simulink model "ModelOfOven"  (R2015a)
settings: Solver=ode3  StartTime=0.0  StopTime=1450  RelTol=1e-3
undefined symbols (not defined in the file or in its folder): sigbuilder_block
libraries: simulink x2, fuzblock x1, sldrtlib x1
settings Model: Creator=Labis Papakostas  LastModifiedBy=Labis Papakostas

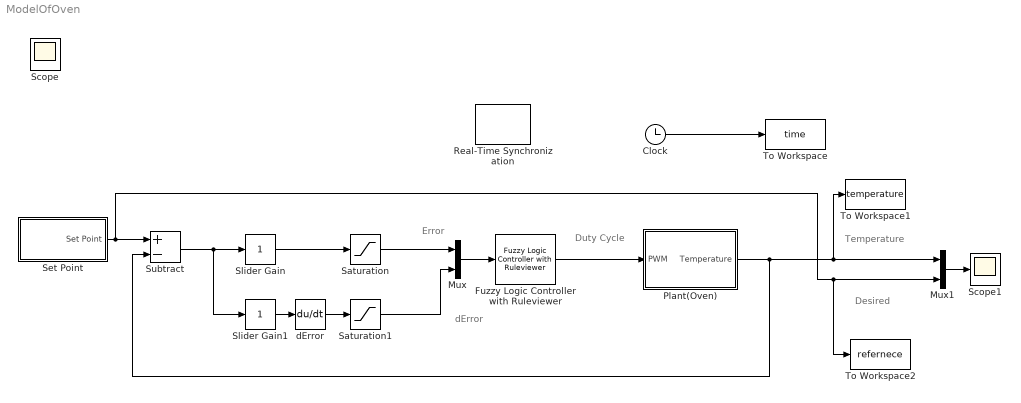
== system ModelOfOven ==
  note: Duty Cycle
  note: dError
  note: Error
  note: Temperature
  note: Desired
  Clock : Clock
  Fuzzy Logic Controller with Ruleviewer : fuzblock/Fuzzy Logic  Controller  with Ruleviewer  fismatrix=Oven  Ts=0.5
  Mux : Mux  Inputs=2
  Mux1 : Mux  Inputs=2
  "Plant(Oven) " : Subsystem
      mask Display: image('Ovenim.jpg')
  Real-Time Synchronization : sldrtlib/Real-Time Synchronization  SampleTime=0.05  MaxMissedTicks=10  ShowMissedTicks=off  YieldWhenWaiting=off
  Saturation : Saturate  UpperLimit=35  LowerLimit=-35
  Saturation1 : Saturate  UpperLimit=35  LowerLimit=-35
  Scope1 : Scope
      settings: YMin=0  YMax=200
  Set Point : Subsystem  Tag=STV Subsys  LoadFcn=sigbuilder_block('load');  StartFcn=sigbuilder_block('start');  StopFcn=sigbuilder_block('stop');  ClipboardFcn=sigbuilder_block('clipboard');  mask(Sigbuilder block){}
      mask help: Simulink:masks:SigbuilderBlock_MD
      mask init:
      | if ~strcmp(get_param(bdroot(gcbh),'SimulationStatus'),'stopped') tuvar = sigbuilder_block('maskInit'); end
      settings: CopyFcn=sigbuilder_block('copy');  DeleteFcn=sigbuilder_block('delete');  ModelCloseFcn=sigbuilder_block('modelClose');  PreSaveFcn=sigbuilder_block('preSave');  PauseFcn=sigbuilder_block('pause');  ContinueFcn=sigbuilder_block('continue');  NameChangeFcn=sigbuilder_block('namechange');  OpenFcn=sigbuilder_block('open',[437.6 199.2 550.4 400 ]);  CloseFcn=sigbuilder_block('close');
      mask Display: plot(0, 0, 100, 100,[2, 2, 32, 32, 2], [68, 8, 8, 68, 68],[32, 2], [38, 38], [32, 19, 2],[53, 60, 44], [32, 17, 17, 2],[16, 16, 31, 31]);txt = getActiveGroup(gcbh);text(2, 100, txt,'verticalAlignment', 'top');
  Slider Gain : simulink/Math Operations/Slider Gain  low=0  gain=1  high=10
  Slider Gain1 : simulink/Math Operations/Slider Gain  low=0  gain=1  high=10
  Subtract : Sum  Inputs=+-
  To Workspace : ToWorkspace  VariableName=time  SampleTime=0.05
      settings: Save2DSignal=2-D array (concatenate along first dimension)
  To Workspace1 : ToWorkspace  VariableName=temperature  SampleTime=0.05
      settings: Save2DSignal=2-D array (concatenate along first dimension)
  To Workspace2 : ToWorkspace  VariableName=refernece  SampleTime=0.05
  dError : Derivative
  Scope : Scope
  wires:
  Subtract/1 -> Slider Gain1/1, Slider Gain/1
  dError/1 -> Saturation1/1
  Mux/1 -> Fuzzy Logic Controller with Ruleviewer/1
  Fuzzy Logic Controller with Ruleviewer/1 -> "Plant(Oven) "/1(PWM)
  Set Point/1(Set Point) -> To Workspace2/1, Mux1/2, Subtract/1
  "Plant(Oven) "/1("Temperature ") -> To Workspace1/1, Mux1/1, Subtract/2
  Slider Gain/1 -> Saturation/1
  Slider Gain1/1 -> dError/1
  Saturation1/1 -> Mux/2
  Saturation/1 -> Mux/1
  Clock/1 -> To Workspace/1
  Mux1/1 -> Scope1/1

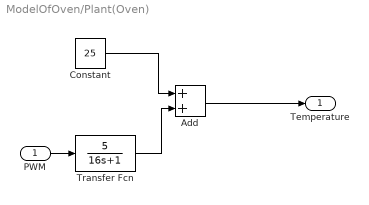
== system ModelOfOven/Plant(Oven)  ==
  PWM : Inport
  Add : Sum
  Constant : Constant  Value=25
  Transfer Fcn : TransferFcn  Numerator=[5]  Denominator=[16 1]
  "Temperature " : Outport
  wires:
  Transfer Fcn/1 -> Add/2
  Add/1 -> "Temperature "/1
  Constant/1 -> Add/1
  PWM/1 -> Transfer Fcn/1

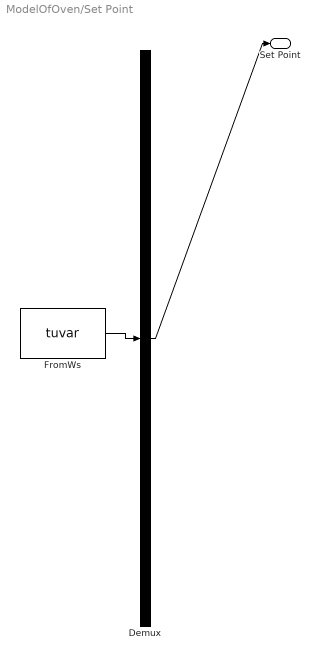
== system ModelOfOven/Set Point ==
  Demux : Demux  Tag=STV Demux  Outputs=1
  FromWs : FromWorkspace  Tag=STV FromWs  VariableName=tuvar  SampleTime=0
      SigBuilderData=|
      | common.afterFinalStr = 'Extrapolate'
      | common.sampleTime = 0
      | dataSet.timeRange = [0 1445]
      | dataSet.name = 'Group 2'
      | sbobj.Groups.Name = 'Group 2'
      | sbobj.Groups.Signals.Name = 'Set Point'
      | sbobj.Groups.Signals.XData = [0 120 120 360 360 480 480 660 660 900 900 1320 1320 1445]
      | sbobj.Groups.Signals.YData = [0 0 180 180 0 0 100 100 0 0 120 120 0 0]
      | sbobj.Groups.TimeRange = [0 1445]
  Set Point : Outport  Tag=STV Outport
  wires:
  FromWs/1 -> Demux/1
  Demux/1 -> Set Point/1
